simulink model "speaker_simulink"  (R2023a)
settings: Solver=VariableStepAuto  StartTime=0.0  StopTime=10  MaxStep=1e-5  RelTol=1e-3  EnableMultiTasking=on
InitFcn:
  | %  Table 10.1 pp 167
  | % MKS units
  | 
  | Re=3.36;              % ohms
  | Le = 0.274e-3;     % henries
  | Bl   = 4.9;              % N/A  Newtons/Amp
  | mm = 14.7e-3;      % kg
  | cm  = 0.56e-3;      % m/N
  | rm  = 0.784;          % kg/s
libraries: dspsrcs4 x1, simulink x1
settings Model: Creator=dbenson  LastModifiedBy=ftiong
settings SolverCC: AlgebraicLoopSolver=TrustRegion
settings DataIOCC: LimitDataPoints=on  SaveFormat=Array  SignalLoggingSaveFormat=ModelDataLogs  ReturnWorkspaceOutputs=off
settings OptimizationCC: ExpressionDepthLimit=2147483647  LifeSpan=inf
settings DebuggingCC: UnderspecifiedInitializationDetection=Classic  MergeDetectMultiDrivingBlocksExec=none  SolverPrmCheckMsg=warning  FcnCallInpInsideContextMsg=warning  UnconnectedInputMsg=warning  UnconnectedOutputMsg=warning  UnconnectedLineMsg=warning  StateNameClashWarn=warning  SFUnexpectedBacktrackingDiag=warning  SFNoUnconditionalDefaultTransitionDiag=warning  SFExecutionAtInitializationDiag=none  ArithmeticOperatorsInVariantConditions=warning
settings HardwareCC: ProdBitPerPointer=32  ProdBitPerSizeT=32  ProdBitPerPtrDiffT=32  ProdLargestAtomicFloat=None  ProdIntDivRoundTo=Undefined  ProdEndianess=Unspecified  ProdWordSize=32  ProdHWDeviceType=32-bit Generic
settings ModelReferenceCC: EnableRefExpFcnMdlSchedulingChecks=on  PropagateSignalLabelsOutOfModel=off
settings SFSimCC: SimUseLocalCustomCode=off  CustomCodeUndefinedFunction=UseInterfaceOnly
settings RTWCC: RTWUseLocalCustomCode=off
settings CodeAppCC: StateflowObjectComments=on
settings GRTTargetCC: TargetLangStandard=C89/C90 (ANSI)  CombineOutputUpdateFcns=off  GRTInterface=on
settings ConfigComp: CovMetricSettings=dw  CovSaveCumulativeToWorkspaceVar=on  CovSaveSingleToWorkspaceVar=on  CovExternalEMLEnable=off  CovSFcnEnable=off
settings SimscapeCC: SimscapeNormalizeSystem=off

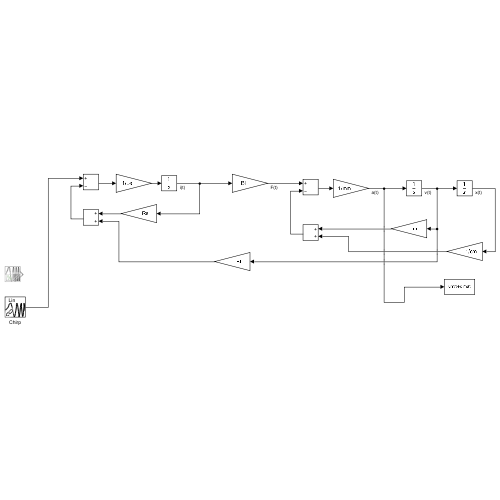
[thumbnail: Simulink's stored preview of the top-level diagram]
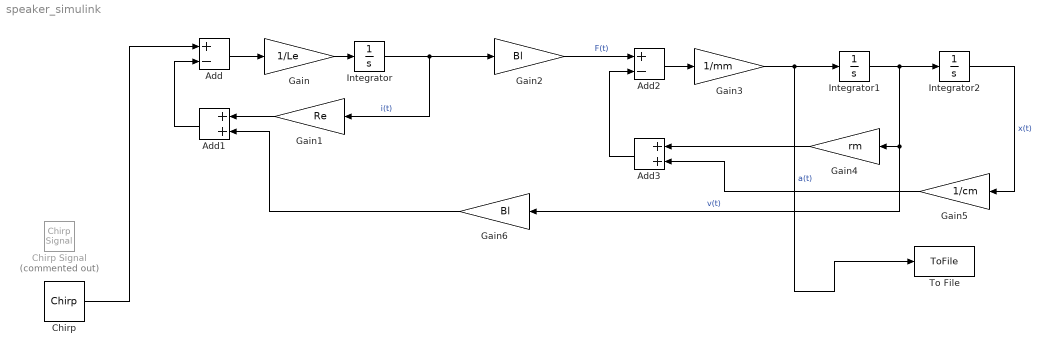
== system speaker_simulink ==
  Add : Sum  Inputs=+-
  Add1 : Sum
  Add2 : Sum  Inputs=+-
  Add3 : Sum
  Chirp : dspsrcs4/Chirp  sweep=Linear  mode=Unidirectional  f0=10  f1=1000  t1=1  Tsweep=1  phase=0  Ts=1/48000  spf=1  datatype=Double  OutputFrames=off
  Chirp Signal : simulink/Sources/Chirp Signal  Commented=on  f1=10  T=1  f2=1000
  Gain : Gain  Gain=1/Le
  Gain1 : Gain  Gain=Re
  Gain2 : Gain  Gain=Bl
  Gain3 : Gain  Gain=1/mm
  Gain4 : Gain  Gain=rm
  Gain5 : Gain  Gain=1/cm
  Gain6 : Gain  Gain=Bl
  Integrator : Integrator
  Integrator1 : Integrator
  Integrator2 : Integrator
  To File : ToFile
  wires:
  Add/1 -> Gain/1
  Gain/1 -> Integrator/1
  Integrator/1 -> Gain2/1, Gain1/1  "i(t)"
  Add1/1 -> Add/2
  Gain1/1 -> Add1/1
  Gain2/1 -> Add2/1  "F(t)"
  Add2/1 -> Gain3/1
  Gain3/1 -> To File/1, Integrator1/1  "a(t)"
  Integrator1/1 -> Integrator2/1, Gain4/1, Gain6/1  "v(t)"
  Integrator2/1 -> Gain5/1  "x(t)"
  Add3/1 -> Add2/2
  Gain4/1 -> Add3/1
  Gain5/1 -> Add3/2
  Gain6/1 -> Add1/2
  Chirp/1 -> Add/1
